simulink model "RootLocusModel"  (R2016b)
settings: Solver=VariableStepAuto  StartTime=0.0  StopTime=30  RelTol=1e-3
values from neighbouring files (symbols this model uses):
  den = [1 0.01 0.0025]    [RootLocusPerformance.m]
  K = 0.74    [RootLocusPerformance.m]
  num = [1 0.2]    [RootLocusPerformance.m]
settings Model: Creator=Christopher  LastModifiedBy=Christopher

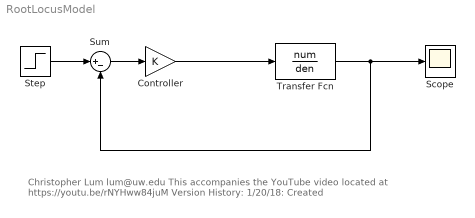
== system RootLocusModel ==
  note: Christopher Lum
      | lum@uw.edu
      |
      | This accompanies the YouTube video located at https://youtu.be/rNYHww84juM
      |
      | Version History:
      | 1/20/18: Created
  Controller : Gain  Gain=K
  Scope : Scope
  Step : Step  SampleTime=0
  Sum : Sum  Inputs=|+-
  Transfer Fcn : TransferFcn  Numerator=num  Denominator=den
  wires:
  Transfer Fcn/1 -> Sum/2, Scope/1
  Controller/1 -> Transfer Fcn/1
  Step/1 -> Sum/1
  Sum/1 -> Controller/1
